simulink model "StateSpaceObserver"  (R2021a)
settings: Solver=FixedStepAuto  StartTime=0.0  StopTime=STime  FixedStep=1e-3  RelTol=1e-3
undefined symbols (not defined in the file): a0, a1, a2, b0, C, dss0, J, K_canobs, Kp, L_obs, Mc, Ra, Ta, Tp, TPert
settings Model: Creator=akangmufti  LastModifiedBy=akangmufti
settings OptimizationCC: DefaultParameterBehavior=Inlined  BufferReuse=off
settings DebuggingCC: InitInArrayFormatMsg=none

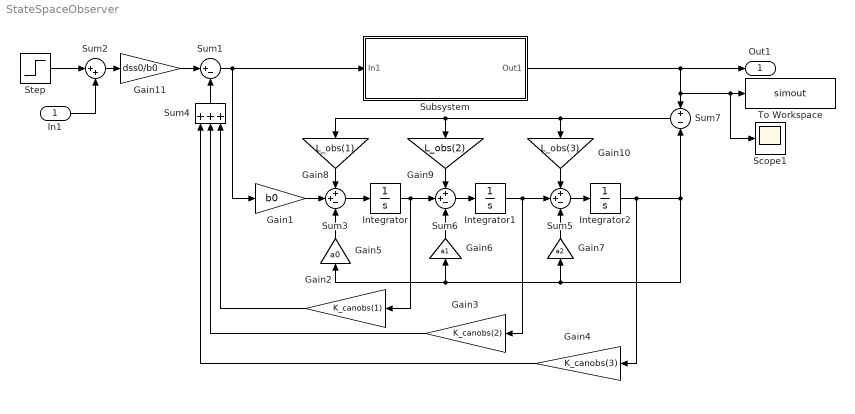
== system StateSpaceObserver ==
  In1 : Inport
  Gain1 : Gain  Gain=b0
  Gain10 : Gain  Gain=L_obs(3)
  Gain11 : Gain  Gain=dss0/b0
  Gain2 : Gain  Gain=K_canobs(1)
  Gain3 : Gain  Gain=K_canobs(2)
  Gain4 : Gain  Gain=K_canobs(3)
  Gain5 : Gain  Gain=a0
  Gain6 : Gain  Gain=a1
  Gain7 : Gain  Gain=a2
  Gain8 : Gain  Gain=L_obs(1)
  Gain9 : Gain  Gain=L_obs(2)
  Integrator : Integrator
  Integrator1 : Integrator
  Integrator2 : Integrator
  Scope1 : Scope
  Step : Step  Time=1e-3  SampleTime=0
  Subsystem : Subsystem
  Sum1 : Sum  Inputs=|+-
  Sum2 : Sum  Inputs=|++
  Sum3 : Sum  Inputs=++-
  Sum4 : Sum  Inputs=+++
  Sum5 : Sum  Inputs=++-
  Sum6 : Sum  Inputs=++-
  Sum7 : Sum  Inputs=+|-
  To Workspace : ToWorkspace  VariableName=simout  SampleTime=-1
  Out1 : Outport
  wires:
  In1/1 -> Sum2/2
  Gain3/1 -> Sum4/2
  Gain4/1 -> Sum4/1
  Gain2/1 -> Sum4/3
  Sum4/1 -> Sum1/2
  Sum3/1 -> Integrator/1
  Sum6/1 -> Integrator1/1
  Gain6/1 -> Sum6/3
  Integrator/1 -> Gain2/1, Sum6/2
  Gain1/1 -> Sum3/2
  Gain5/1 -> Sum3/3
  Gain7/1 -> Sum5/3
  Gain9/1 -> Sum6/1
  Gain8/1 -> Sum3/1
  Gain10/1 -> Sum5/1
  Sum5/1 -> Integrator2/1
  Integrator2/1 -> Gain4/1, Sum7/2, Gain5/1, Gain6/1, Gain7/1
  Integrator1/1 -> Gain3/1, Sum5/2
  Step/1 -> Sum2/1
  Sum1/1 -> Gain1/1, Subsystem/1(In1)
  Sum7/1 -> Gain10/1, Gain8/1, Gain9/1
  Sum2/1 -> Gain11/1
  Subsystem/1(Out1) -> Scope1/1, To Workspace/1, Sum7/1, Out1/1
  Gain11/1 -> Sum1/1

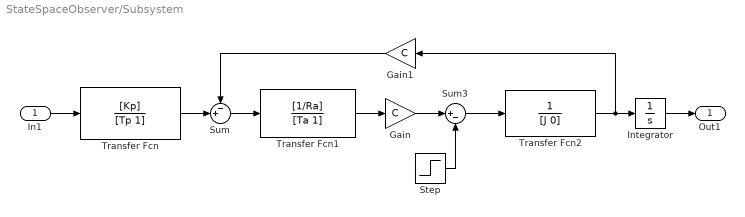
== system StateSpaceObserver/Subsystem ==
  In1 : Inport
  Gain : Gain  Gain=C
  Gain1 : Gain  Gain=C
  Integrator : Integrator
  Step : Step  Time=TPert  After=Mc  SampleTime=0
  Sum : Sum  Inputs=-+|
  Sum3 : Sum  Inputs=|+-
  Transfer Fcn : TransferFcn  Numerator=[Kp]  Denominator=[Tp 1]
  Transfer Fcn1 : TransferFcn  Numerator=[1/Ra]  Denominator=[Ta 1]
  Transfer Fcn2 : TransferFcn  Denominator=[J 0]
  Out1 : Outport
  wires:
  Transfer Fcn1/1 -> Gain/1
  Gain/1 -> Sum3/1
  Sum/1 -> Transfer Fcn1/1
  Sum3/1 -> Transfer Fcn2/1
  Gain1/1 -> Sum/1
  Transfer Fcn2/1 -> Integrator/1, Gain1/1
  Step/1 -> Sum3/2
  Transfer Fcn/1 -> Sum/2
  In1/1 -> Transfer Fcn/1
  Integrator/1 -> Out1/1
